simulink model "model_mod_reg_nabl"  (R2021b)
settings: Solver=FixedStepAuto  StartTime=0.0  StopTime=2.5  FixedStep=Ts  RelTol=1e-3
values from neighbouring files (symbols this model uses):
  Kd = place(SYS.A,SYS.B,pd)    [vipolnenie_lr_3.m]
  kdnorm = ydu/yduk    [vipolnenie_lr_3.m]
  L = l'    [vipolnenie_lr_3.m]
  SYS = ss(a,b,c,d,Ts)    [vipolnenie_lr_3.m]
  Ts = 0.01    [vipolnenie_lr_3.m]
settings Model: Creator=Admin  LastModifiedBy=Admin
settings SolverCC: AlgebraicLoopSolver=TrustRegion
settings DebuggingCC: ArithmeticOperatorsInVariantConditions=warning
settings SFSimCC: CustomCodeUndefinedFunction=UseInterfaceOnly

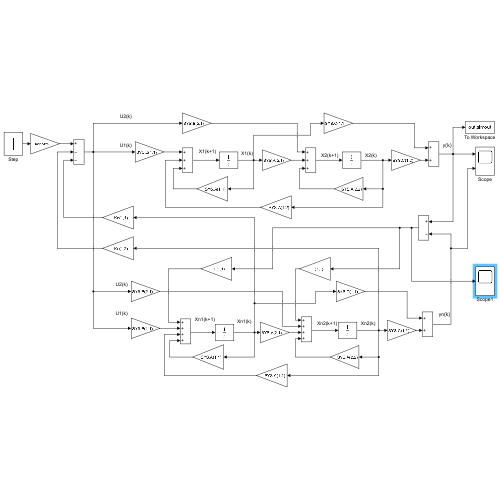
[thumbnail: Simulink's stored preview of the top-level diagram]
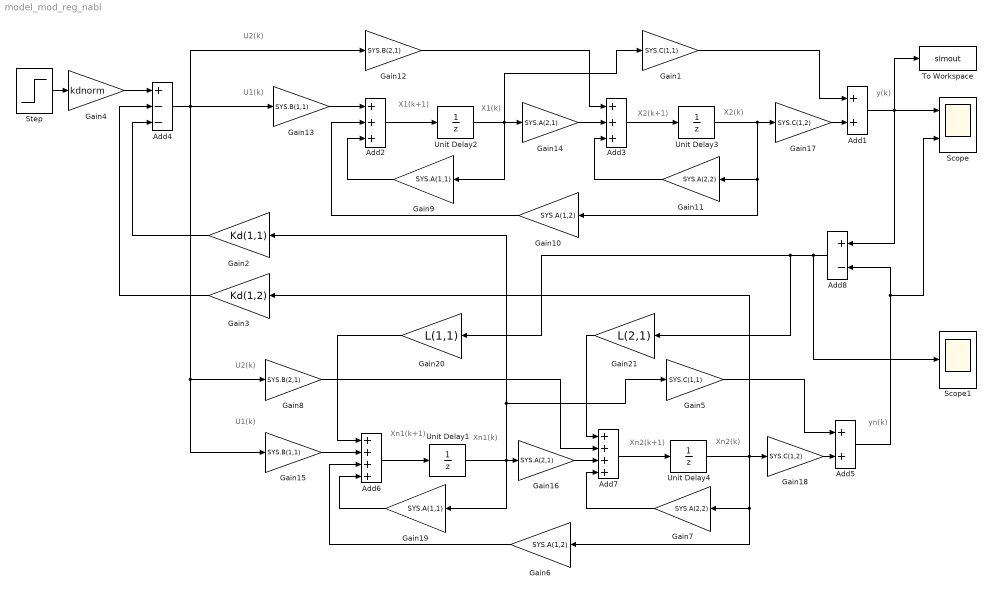
== system model_mod_reg_nabl ==
  note: y(k)
  note: X2(k)
  note: X2(k+1)
  note: X1(k)
  note: U2(k)
  note: X1(k+1)
  note: U1(k)
  note: U2(k)
  note: Xn1(k+1)
  note: yn(k)
  note: U1(k)
  note: Xn2(k)
  note: Xn1(k)
  note: Xn2(k+1)
  Add1 : Sum
  Add2 : Sum  Inputs=+++
  Add3 : Sum  Inputs=+++
  Add4 : Sum  Inputs=+--
  Add5 : Sum
  Add6 : Sum  Inputs=++++
  Add7 : Sum  Inputs=++++
  Add8 : Sum  Inputs=+-
  Gain1 : Gain  Gain=SYS.C(1,1)
  Gain10 : Gain  Gain=SYS.A(1,2)
  Gain11 : Gain  Gain=SYS.A(2,2)
  Gain12 : Gain  Gain=SYS.B(2,1)
  Gain13 : Gain  Gain=SYS.B(1,1)
  Gain14 : Gain  Gain=SYS.A(2,1)
  Gain15 : Gain  Gain=SYS.B(1,1)
  Gain16 : Gain  Gain=SYS.A(2,1)
  Gain17 : Gain  Gain=SYS.C(1,2)
  Gain18 : Gain  Gain=SYS.C(1,2)
  Gain19 : Gain  Gain=SYS.A(1,1)
  Gain2 : Gain  Gain=Kd(1,1)
  Gain20 : Gain  Gain=L(1,1)
  Gain21 : Gain  Gain=L(2,1)
  Gain3 : Gain  Gain=Kd(1,2)
  Gain4 : Gain  Gain=kdnorm
  Gain5 : Gain  Gain=SYS.C(1,1)
  Gain6 : Gain  Gain=SYS.A(1,2)
  Gain7 : Gain  Gain=SYS.A(2,2)
  Gain8 : Gain  Gain=SYS.B(2,1)
  Gain9 : Gain  Gain=SYS.A(1,1)
  Scope : Scope  NumInputPorts=2
  Scope1 : Scope
  Step : Step  Time=0  SampleTime=0
  To Workspace : ToWorkspace  VariableName=simout  SaveFormat=Timeseries  SampleTime=-1
  Unit Delay{1..4} (4 alike) : UnitDelay  SampleTime=Ts  HasFrameUpgradeWarning=on
  wires:
  Gain1/1 -> Add1/1
  Gain17/1 -> Add1/2
  Add1/1 -> To Workspace/1, Scope/1, Add8/1
  Gain11/1 -> Add3/3
  Gain9/1 -> Add2/3
  Unit Delay2/1 -> Gain9/1, Gain1/1, Gain14/1
  Gain14/1 -> Add3/2
  Add2/1 -> Unit Delay2/1
  Gain13/1 -> Add2/1
  Add3/1 -> Unit Delay3/1
  Gain10/1 -> Add2/2
  Unit Delay3/1 -> Gain11/1, Gain10/1, Gain17/1
  Gain12/1 -> Add3/1
  Add4/1 -> Gain12/1, Gain15/1, Gain8/1, Gain13/1
  Gain2/1 -> Add4/3
  Gain3/1 -> Add4/2
  Gain4/1 -> Add4/1
  Step/1 -> Gain4/1
  Unit Delay4/1 -> Gain3/1, Gain18/1, Gain7/1, Gain6/1
  Add7/1 -> Unit Delay4/1
  Add6/1 -> Unit Delay1/1
  Gain18/1 -> Add5/2
  Unit Delay1/1 -> Gain2/1, Gain5/1, Gain19/1, Gain16/1
  Gain5/1 -> Add5/1
  Add5/1 -> Add8/2, Scope/2
  Gain19/1 -> Add6/4
  Gain6/1 -> Add6/3
  Gain15/1 -> Add6/2
  Gain20/1 -> Add6/1
  Gain7/1 -> Add7/4
  Gain16/1 -> Add7/3
  Gain8/1 -> Add7/2
  Gain21/1 -> Add7/1
  Add8/1 -> Scope1/1, Gain21/1, Gain20/1
